simulink model "video_model"  (R2018b)
settings: Solver=FixedStepDiscrete  StartTime=0.0  StopTime=inf  RelTol=1e-3
values from neighbouring files (symbols this model uses):
  model_skory = createSkinModel2(RGB,BW)    [createProbabilityImage.m]    (also in dane_modelu.mat = [0 0 0 0 0 0 0 0 0 0 0 0 ... (65536 elements, 256x256)])
undefined symbols (not defined in the file or in its folder): Rec, SDTV
libraries: visionconversions x1, dspvision x1
settings Model: Creator=marek  LastModifiedBy=marek

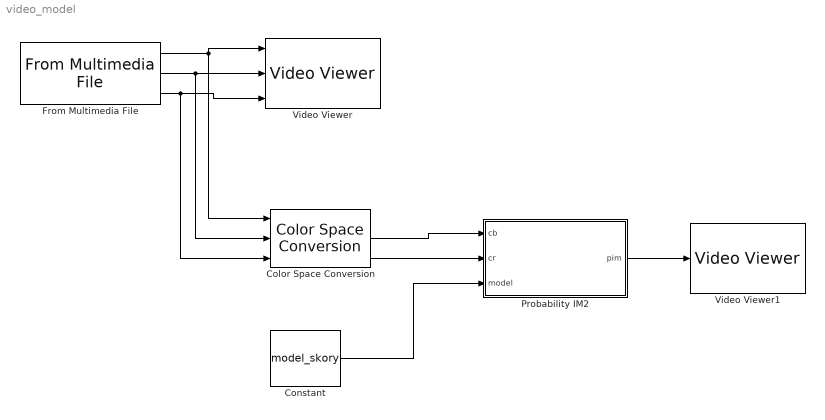
== system video_model ==
  Color Space Conversion : visionconversions/Color Space  Conversion  conversion=Obsolete  conversionActive=R'G'B' to Y'CbCr  wp_str=D65  rec=Rec. 601 (SDTV)  sys=1125/60/2:1  imagePorts=Separate color signals
      settings: SourceProductName=Computer Vision System Toolbox
  Constant : Constant  Value=model_skory
  From Multimedia File : dspvision/From Multimedia File  inputFilename=video_material.avi  loop=on  numPlays=inf  outputStreams=Video only  videoDataType=uint8  audioDataType=int16  inheritSampleTime=on  userDefinedSampleTime=1/30  noAudioOutput=off  isIntensityVideo=off  fourcc=RGB  colorVideoFormat=Separate color signals  outputEOF=off  dataOrg=Column-major  audioFrameSize=1024  computeAudioFrameSize=off  outSamplingMode=Sample based
      settings: SourceProductBaseCode=VP
  Probability IM2 : MATLAB Function  TreatAsAtomicUnit=on
  Video Viewer : VideoViewer  imagePorts=separate color signals  FigPos=[534.6 606.8 417.6 304]
  Video Viewer1 : VideoViewer  FigPos=[559 583 418 304]
  wires:
  From Multimedia File/1 -> Color Space Conversion/1, Video Viewer/1
  From Multimedia File/2 -> Color Space Conversion/2, Video Viewer/2
  From Multimedia File/3 -> Color Space Conversion/3, Video Viewer/3
  Color Space Conversion/2 -> Probability IM2/1(cb)
  Color Space Conversion/3 -> Probability IM2/2(cr)
  Constant/1 -> Probability IM2/3(model)
  Probability IM2/1(pim) -> Video Viewer1/1

== matlab function video_model/Probability IM2 ==
  data: cb input; cr input; model input; pim output
function pim = probabilityIM2(cb,cr,model)
%#codegen
% Wyznaczenie tablicy prawdopodobienstwa dla obrazu wg zadanego modelu koloru skory.
%
% INPUT:
% > im - testowy obraz wejsciowy w formacie RGB
% > model - model koloru skory (tablica [256*256])
% OUTPUT:                                                                         
% > skin_model - obraz prawdopodobienstwa
%
% DEPENDICIES:
% -
% COMMENTS:
% > Wykorzystano przeksztalcenie look-up-table 2D
% > TODO kontrola argumentow wejsciowych
% CREATED: Jaromir Przybylo, 26.10.2015, R2015a
% LASTMODIFIED: 
%

ind=sub2ind([256 256],cb(:),cr(:));
outim=model(ind);
pim=reshape(outim,size(cb(:,:,1)));
